simulink model "Sailboat_Modeling"  (R2024a)
settings: Solver=VariableStepAuto  StartTime=0.0  StopTime=10.0  RelTol=1e-3
values from neighbouring files (symbols this model uses):
  Ixx = 1/120 * pi * rho * L * B * T * (4*T^2 + B^2)    (= 0.835683076278)    [parameterCalculations.m]
  Izz = 1/120 * pi * rho * L * B * T * (B^2 + L^2)    (= 1.17027496573)    [parameterCalculations.m]
  m = 2.7    [parameterCalculations.m]
  m11 = m*k11    [parameterCalculations.m]
  m22 = m*k22    [parameterCalculations.m]
  m24 = 0    [parameterCalculations.m]
  m26 = xb*m22    [parameterCalculations.m]
  m66 = k66*Izz    [parameterCalculations.m]
  Nr = -pi * T^2/L^2 * (0.25 +0.039 * B/T - 0.56 * B/L)    (= -0.104988463049)    [parameterCalculations.m]
  Nv = -pi * T^2/L^2 * (0.5 +2.4 * T/L)    (= -0.841300100031)    [parameterCalculations.m]
  Yv = -pi * T^2/L^2 * (1 +0.4 * CB * B/T)    (= -0.560439243466)    [parameterCalculations.m]
libraries: cstblocks x4, simulink x3, vrlib x1
settings Model: Creator=Ruben  LastModifiedBy=Ruben

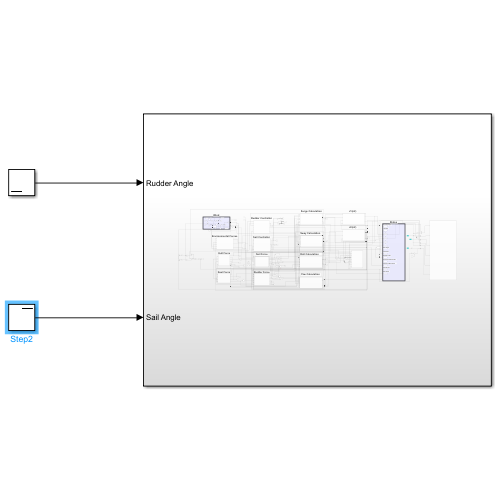
[thumbnail: Simulink's stored preview of the top-level diagram]
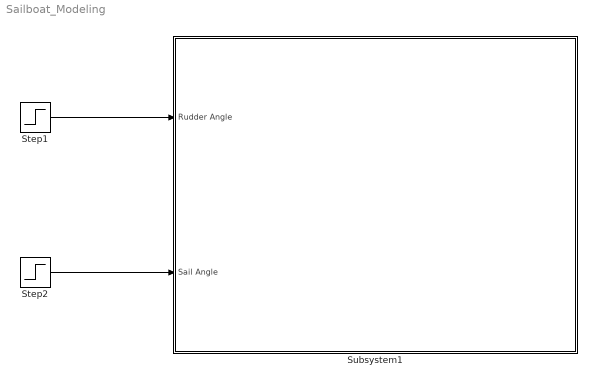
== system Sailboat_Modeling ==
  Step1 : Step  Time=0  After=0  SampleTime=0
  Step2 : Step  Time=0  After=pi/4  SampleTime=0
  Subsystem1 : Subsystem
  wires:
  Step2/1 -> Subsystem1/2(Sail Angle)
  Step1/1 -> Subsystem1/1(Rudder Angle)

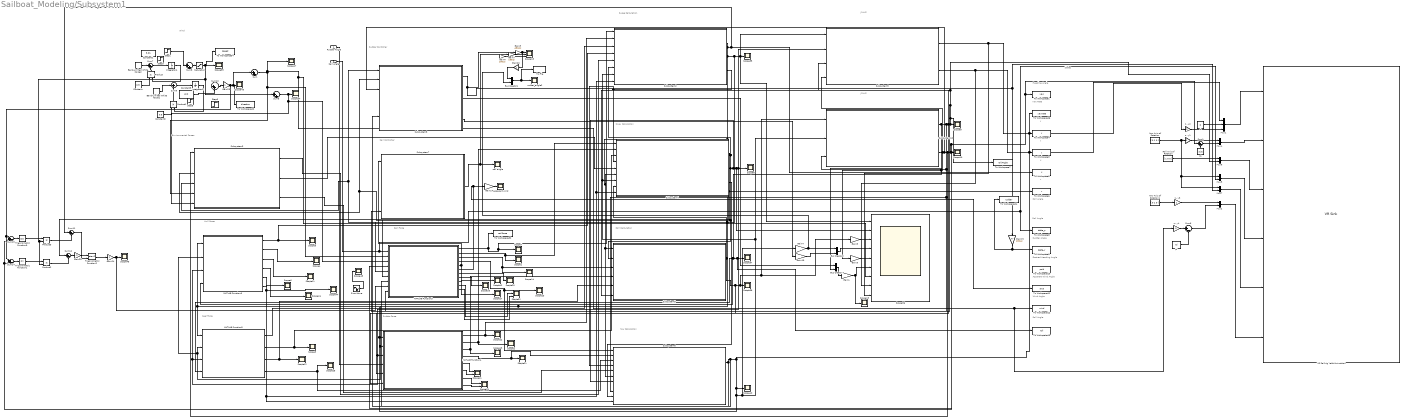
== system Sailboat_Modeling/Subsystem1 ==
  note: Keel Force
  note: Rudder Force
  note: Wind
  note: Sway Calculation
  note: Desired Heading Angle
  note: Sail Force
  note: u
  note: Environmental Forces
  note: J1(n2)
  note: Rudder Angle
  note: Apparent Wind Angle
  note: Yaw Calculation
  note: y
  note: v
  note: Surge Calculation
  note: Rudder Controller
  note: Wind Angle
  note: x
  note: States
  note: Heading Angle
  note: Sail Angle
  note: J2(n2)
  note: Sail Controller
  note: Yaw Rate
  note: Hull Force
  note: Roll Calculation
  note: Roll Angle
  note: Roll Angle
  Rudder Angle : Inport
  Sail Angle : Inport  Port=2
  Band-Limited White Noise1 : simulink/Sources/Band-Limited White Noise  Cov=[0.225]  Ts=0.01  seed=[3341]
  Band-Limited White Noise2 : simulink/Sources/Band-Limited White Noise  Cov=[0.2]  Ts=0.01  seed=[23341]
  Bus Creator : BusCreator  Inputs=2
  Bus Creator1 : BusCreator  Inputs=2
  Bus Creator2 : BusCreator  Inputs=2
  Constant : Constant  Value=0.5
  Constant1 : Constant  Value=3.01
  Constant2 : Constant  Value=0.5
  Constant3 : Constant  Value=pi/2
  Gain{1,3..7,14,18..19} (9 alike) : Gain  Gain=180/pi
  Gain20 : Gain
  Gain23 : Gain
  Gain24 : Gain
  Gain25 : Gain  Gain=-1
  Gain8 : Gain  Gain=-180/pi
  Integrator2 : Integrator  LimitOutput=on  UpperSaturationLimit=99  LowerSaturationLimit=-99
  Integrator4 : Integrator
  MATLAB Function3 : MATLAB Function  TreatAsAtomicUnit=on
  MATLAB Function4 : MATLAB Function  TreatAsAtomicUnit=on
  MATLAB Function5 : MATLAB Function  TreatAsAtomicUnit=on
  MATLAB Function6 : MATLAB Function  TreatAsAtomicUnit=on
  Mux1 : Mux  Inputs=3
  Mux{2,4..7} (5 alike) : Mux  Inputs=2
  Product{,1..3} (4 alike) : Product
  Roll Axis of Rotation : Constant  Value=[ 1 0 0 ]
  Saturation : Saturate  UpperLimit=6  LowerLimit=0
  Scope{1..14,17,19..27,34..35,37..40,42..45,48} (35 alike) : Scope
  Scope15 : Scope  NumInputPorts=3
  Scope31 : Scope  NumInputPorts=2
  Scope32 : Scope  NumInputPorts=2
  Scope36 : Scope  NumInputPorts=9
  Scope41 : Scope  NumInputPorts=2
  Sine Wave : Sin  Amplitude=pi  SampleTime=0
  Step1 : Step  Time=0  After=2  SampleTime=0
  Step3 : Step  Time=10  After=0.5  SampleTime=0
  Step5 : Step  Time=40  After=0.5  SampleTime=0
  Step6 : Step  Time=30  After=0.5  SampleTime=0
  Subsystem10 : Subsystem
  Subsystem2 : Subsystem
  Subsystem3 : Subsystem
  Subsystem4 : Subsystem
  Subsystem5 : Subsystem
  Subsystem6 : Subsystem
  Subsystem7 : Subsystem
  Subsystem8 : Subsystem
  Subsystem9 : Subsystem
  Sum{,5,8,10} (4 alike) : Sum  Inputs=|++
  Sum1 : Sum  Inputs=|+-  SaturateOnIntegerOverflow=on
  Sum{6..7,9,11..12} (5 alike) : Sum  Inputs=|+-
  Sum13 : Sum  Inputs=|-+-
  Sum14 : Sum  Inputs=|-+-
  To File : ToFile  Filename=sim_step.mat  SaveFormat=Timeseries
  To Workspace1 : ToWorkspace  VariableName=yaw  SaveFormat=Timeseries  SampleTime=0.01
  To Workspace10 : ToWorkspace  VariableName=psid  SaveFormat=Timeseries  SampleTime=0.01
  To Workspace11 : ToWorkspace  VariableName=awa  SaveFormat=Timeseries  SampleTime=-1
  To Workspace12 : ToWorkspace  VariableName=wind  SaveFormat=Timeseries  SampleTime=-1
  To Workspace13 : ToWorkspace  VariableName=roll  SaveFormat=Timeseries  SampleTime=-1
  To Workspace22 : ToWorkspace  VariableName=direction  SaveFormat=Timeseries  SampleTime=-1
  To Workspace24 : ToWorkspace  VariableName=rudder  SaveFormat=Timeseries  SampleTime=0.01
  To Workspace26 : ToWorkspace  VariableName=yawrate  SaveFormat=Timeseries  SampleTime=0.01
  To Workspace3 : ToWorkspace  VariableName=x  SaveFormat=Timeseries  SampleTime=-1
  To Workspace32 : ToWorkspace  VariableName=sailforce  SaveFormat=Timeseries  SampleTime=0.01
  To Workspace34 : ToWorkspace  VariableName=speed  SaveFormat=Timeseries  SampleTime=0.01
  To Workspace4 : ToWorkspace  VariableName=y  SaveFormat=Timeseries  SampleTime=-1
  To Workspace5 : ToWorkspace  VariableName=u  SaveFormat=Timeseries  SampleTime=0.01
  To Workspace6 : ToWorkspace  VariableName=v  SaveFormat=Timeseries  SampleTime=-1
  To Workspace7 : ToWorkspace  VariableName=rollAngle  SaveFormat=Timeseries  SampleTime=0.01
  To Workspace8 : ToWorkspace  VariableName=delta_s  SaveFormat=Timeseries  SampleTime=-1
  To Workspace9 : ToWorkspace  VariableName=delta_r  SaveFormat=Timeseries  SampleTime=0.01
  Trigonometric Function1 : Trigonometry
  Trigonometric Function2 : Trigonometry  Operator=atan2
  Trigonometric Function9 : Trigonometry  Operator=cos
  VR Sailing Yacht Animation : vrlib/VR Sink  InstantiateOnLoad=on  SampleTime=0.05  ViewEnable=on  RemoteChange=off  RemoteView=off  FieldsWritten=Hull_EarthFixed.translation.3.1.1.double#Rot_Yaw.rotation.4.1.1.double#Rot_Roll.rotation.4.1.1.double#Sail.rotation.4.1.1.double#Rudder.rotation.4.1.1.double#Wind_Arrow.rotation.4.1.1.double  WorldFileName=SailingYachtAnimation.wrl  WorldDescription=Sailing Yacht VR animation  AutoView=on  VideoDimensions=[]  AllowVariableSize=off  FigureProperties="{'Position', 'Name', 'Viewpoint', 'CameraBound', 'CameraDirection', 'CameraPosition', 'CameraUpVector', 'ZoomFactor', 'Antialiasing', 'Headlight', 'Lighting', 'Sound', 'StatusBar', 'Stereo3D', 'Stereo3DCameraOffset', 'Stereo3DHIT', 'ToolBar', 'Textures', 'Transparency', 'Triad', 'Wireframe', 'NavZones', 'NavMode', 'NavSpeed', 'CaptureFileFormat', 'CaptureFileName', 'Record2DCompressMethod', 'Record2DCompressQuality', 'Record2D', 'Record2DFileName', 'Record2DFPS', 'NavPanel'; [9.6200000000000000e+02   8.4000000000000000e+01   9.5800000000000000e+02   3.8000000000000000e+02], 'Sailing Yacht VR animation', 'Stern', 'on', [1.8779174371111376e-01  -8.0146307062595545e-01  -5.6779503997195024e-01], [-1.3398952830018864e+01   3.3896676016628582e+01   3.0405778585208221e+01], [8.9478754028877491e-02   5.8963553407129154e-01  -8.0269763269733285e-01], [1.0000000000000000e+00], 'on', 'on', 'on', 'on', 'on', 'off', [1.0000000149011612e-01], [0.0000000000000000e+00], 'on', 'on', 'on', 'none', 'off', 'off', 'fly', 'normal', 'tif', '%f_anim_%n.tif', 'auto', [7.5000000000000000e+01], 'off', '%f_anim_%n.avi', 'auto', 'halfbar'}"
  Yaw Axis of Rotation : Constant  Value=[ 0 1 0 ]
  Yaw Axis of Rotation1 : Constant  Value=[ 0 1 0 ]
  apparent wind : Scope
  pi : Constant  Value=-pi
  rudder_angle2 : Scope
  sail angle : Scope
  z : Constant  Value=0
  z - y1 : Gain
  z - y2 : Gain  Gain=-1
  z - y3 : Gain
  z - y4 : Gain  Gain=-1
  z1 : Constant  Value=pi/2
  wires:
  Step1/1 -> Sum8/1
  Bus Creator2/1 -> Scope36/4
  MATLAB Function3/2(Ys) -> Scope1/1, Subsystem4/1(sail force (Ys))
  Constant2/1 -> Product1/1
  Subsystem10/1(Phi) -> Gain3/1, MATLAB Function5/4(phi), MATLAB Function6/4(phi), To Workspace13/1, Scope37/1, Subsystem6/9(roll), Subsystem7/4(roll_angle), Subsystem10/3(phi), MATLAB Function4/6(phi), Subsystem9/3(phi), Scope9/1, To Workspace7/1, MATLAB Function3/9(phi), Subsystem5/6(rudder force (Kr)), Mux6/2
  Subsystem8/2(Desired Heading) -> Bus Creator/1
  Bus Creator1/1 -> To File/1, rudder_angle2/1
  Gain20/1 -> Bus Creator1/1
  Sum10/1 -> Gain23/1
  MATLAB Function6/1(Xh) -> Scope5/1, Subsystem2/4(hull force (Xh))
  MATLAB Function3/1(Xs) -> Subsystem2/1(sail force (Xs)), Scope7/1, To Workspace32/1
  MATLAB Function4/4(Nr) -> Scope21/1, Subsystem6/2(rudder force (Nr))
  MATLAB Function3/11(D) -> Scope32/2
  Subsystem7/1(sail angle) -> Gain7/1, sail angle/1
  Gain8/1 -> Gain20/1, Scope15/1
  Subsystem6/1(r) -> Subsystem8/6(r), To Workspace26/1, MATLAB Function5/1(r), MATLAB Function6/1(r), MATLAB Function4/1(r), Gain4/1, Subsystem10/2(r), Subsystem2/7(r), Subsystem4/7(r), Scope40/1, MATLAB Function3/7(r)
  MATLAB Function3/5(awa) -> Scope42/1, Subsystem7/1(apparent_wind_angle)
  MATLAB Function3/7(apparent_velocity) -> Scope20/1
  Gain19/1 -> Bus Creator2/2
  Subsystem8/3(desired yaw rate) -> Gain19/1
  Gain7/1 -> Scope15/2
  Gain1/1 -> Scope19/1, Scope36/6
  MATLAB Function5/2(Yk) -> Scope3/1, Subsystem4/3(keel force (Yk))
  MATLAB Function5/1(Xk) -> Subsystem2/3(keel force (Xk))
  Sum5/1 -> Scope34/1, Subsystem3/6(wind Velocity), MATLAB Function3/3(wind_velocity)
  Gain6/1 -> Scope15/3
  z/1 -> Mux1/2
  MATLAB Function4/7(lift_force) -> Scope31/1
  MATLAB Function3/10(L) -> Scope32/1
  Mux1/1 -> VR Sailing Yacht Animation/1
  Subsystem3/3(Ne) -> Subsystem6/5(environmental force (Ne))
  MATLAB Function3/9(V_awv) -> Scope27/1
  Subsystem4/2(v dot) -> Subsystem6/10(vdot)
  MATLAB Function3/8(V_awu) -> Scope26/1
  Subsystem9/1(x) -> Scope36/9, z - y2/1, To Workspace4/1
  MATLAB Function4/5(delta_r) -> Scope41/1
  MATLAB Function3/6(alpha_aw) -> To Workspace11/1, Gain14/1
  z1/1 -> Sum1/2
  MATLAB Function4/2(Yr) -> Scope2/1, Subsystem4/2(rudder force (Yr))
  Gain4/1 -> Bus Creator2/1, Bus Creator1/2
  Gain18/1 -> To Workspace9/1, To Workspace24/1
  MATLAB Function6/3(Kh) -> Scope11/1
  MATLAB Function3/3(Ks) -> Scope14/1, Subsystem5/3(sail force (Ks))
  MATLAB Function5/4(Nk) -> Scope25/1, Subsystem6/3(keel force (Nk))
  MATLAB Function4/3(Kr) -> Scope13/1, Subsystem5/4(roll angle)
  MATLAB Function5/3(Kk) -> Scope12/1, Subsystem5/5(keel force (Kk))
  Subsystem4/1(v) -> To Workspace6/1, MATLAB Function3/6(v), Subsystem2/6(v), Subsystem6/7(v), Scope36/2, Scope8/1, Subsystem9/2(v), MATLAB Function6/3(v), MATLAB Function5/3(v), MATLAB Function4/3(v), Subsystem5/2(v), Subsystem8/2(v), Subsystem3/3(v), Sum12/1
  MATLAB Function4/1(Xr) -> Subsystem2/2(rudder force (Xr)), Scope22/1
  Mux6/1 -> VR Sailing Yacht Animation/3
  Subsystem3/2(Ye) -> Subsystem4/5(environmental force (Ye))
  Subsystem3/1(Xe) -> Subsystem2/5(environmental force (Xe))
  Mux7/1 -> VR Sailing Yacht Animation/5
  Sine Wave/1 -> Scope48/1
  Subsystem10/2(Psi) -> Bus Creator/2, Subsystem9/4(psi), Sum14/2, Sum13/2, Sum1/1, To Workspace1/1, MATLAB Function3/4(psi), Scope10/1, Subsystem3/1(psi), Subsystem8/3(psi)
  Yaw Axis of Rotation/1 -> Mux5/1, Mux7/1, z - y1/1
  Constant3/1 -> Sum10/2
  z - y4/1 -> Sum6/1
  MATLAB Function6/4(Nh) -> Scope24/1
  MATLAB Function4/6(alpha_a) -> Scope41/2
  z - y3/1 -> Mux2/1
  Subsystem8/1(rudder angle) -> Gain8/1, Gain18/1, Mux7/2
  Subsystem5/1(p) -> MATLAB Function4/5(p), Subsystem10/1(p), Gain5/1, Scope38/1, Subsystem4/8(p)
  Saturation/1 -> Product2/2, Product3/2, Sum5/1, Scope39/1, To Workspace34/1
  MATLAB Function4/8(drag_force) -> Scope31/2
  Sum6/1 -> Mux2/2
  MATLAB Function6/2(Yh) -> Scope4/1
  Integrator2/1 -> Product1/2
  Band-Limited White Noise1/1 -> Sum9/1
  MATLAB Function3/4(Ns) -> Subsystem6/1(sail force (Ns)), Scope23/1
  Integrator4/1 -> Product/2
  MATLAB Function6/6(alpha_ah) -> Subsystem6/11(hull_ah), Subsystem2/8(hull_ah), Subsystem4/9(hull_ah), Scope44/1
  Sum/1 -> Scope17/1, Scope36/7, z - y4/1, To Workspace12/1, MATLAB Function3/2(wind_direction), Subsystem3/5(wind Direction)
  Product1/1 -> Sum9/2
  Band-Limited White Noise2/1 -> Sum7/1
  Product/1 -> Sum7/2
  Subsystem2/1(u) -> MATLAB Function5/2(u), MATLAB Function6/2(u), MATLAB Function4/2(u), Subsystem8/1(u), Subsystem3/4(u), Subsystem6/6(u), Subsystem5/1(u), Subsystem4/6(u), MATLAB Function3/5(u), Scope36/1, Subsystem9/1(u), Scope35/1, Sum11/1, To Workspace5/1
  Sum7/1 -> Integrator4/1
  z - y1/1 -> Mux4/1
  pi/1 -> Sum6/2
  Sum9/1 -> Integrator2/1
  Mux4/1 -> VR Sailing Yacht Animation/2
  Bus Creator/1 -> Gain1/1
  Gain14/1 -> apparent wind/1
  Gain5/1 -> Scope36/3
  Constant/1 -> Product/1
  Gain23/1 -> Sum14/1, Sum13/1, Sum/1, To Workspace22/1, Scope43/1
  Subsystem9/2(y) -> Scope36/8, Mux1/1, To Workspace3/1
  Subsystem2/2(hull) -> Subsystem6/4(hull force (Nh)), Subsystem4/4("hull force ")
  Yaw Axis of Rotation1/1 -> z - y3/1
  MATLAB Function6/5(Frh) -> Scope6/1
  Sum1/1 -> Mux4/2
  Gain3/1 -> Scope36/5
  Mux5/1 -> VR Sailing Yacht Animation/4
  Sum8/1 -> Saturation/1
  Mux2/1 -> VR Sailing Yacht Animation/6
  Roll Axis of Rotation/1 -> Mux6/1
  z - y2/1 -> Mux1/3
  Rudder Angle/1 -> MATLAB Function4/4("delta_r ")
  Product2/1 -> Sum12/2
  Gain25/1 -> Trigonometric Function2/1
  Gain24/1 -> MATLAB Function3/8(rawa), Scope45/1
  Sum12/1 -> Gain25/1
  Sum13/1 -> Trigonometric Function9/1
  Sum14/1 -> Trigonometric Function1/1
  Product3/1 -> Sum11/2
  Trigonometric Function1/1 -> Product2/1
  Trigonometric Function9/1 -> Product3/1
  Trigonometric Function2/1 -> Gain24/1
  Sum11/1 -> Trigonometric Function2/2
  Sail Angle/1 -> To Workspace8/1, Mux5/2, MATLAB Function3/1(delta_s)

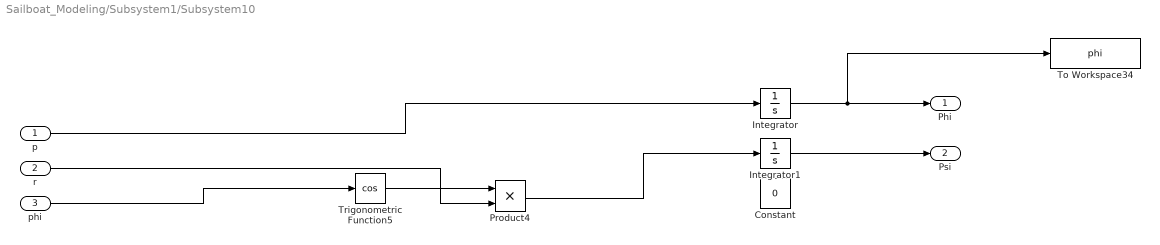
== system Sailboat_Modeling/Subsystem1/Subsystem10 ==
  p : Inport
  r : Inport  Port=2
  phi : Inport  Port=3
  Constant : Constant  Value=0
  Integrator : Integrator
  Integrator1 : Integrator
  Product4 : Product
  To Workspace34 : ToWorkspace  VariableName=phi  SaveFormat=Timeseries  SampleTime=0.01
  Trigonometric Function5 : Trigonometry  Operator=cos
  Phi : Outport
  Psi : Outport  Port=2
  wires:
  Integrator/1 -> To Workspace34/1, Phi/1
  p/1 -> Integrator/1
  Trigonometric Function5/1 -> Product4/1
  Product4/1 -> Integrator1/1
  r/1 -> Product4/2
  phi/1 -> Trigonometric Function5/1
  Integrator1/1 -> Psi/1

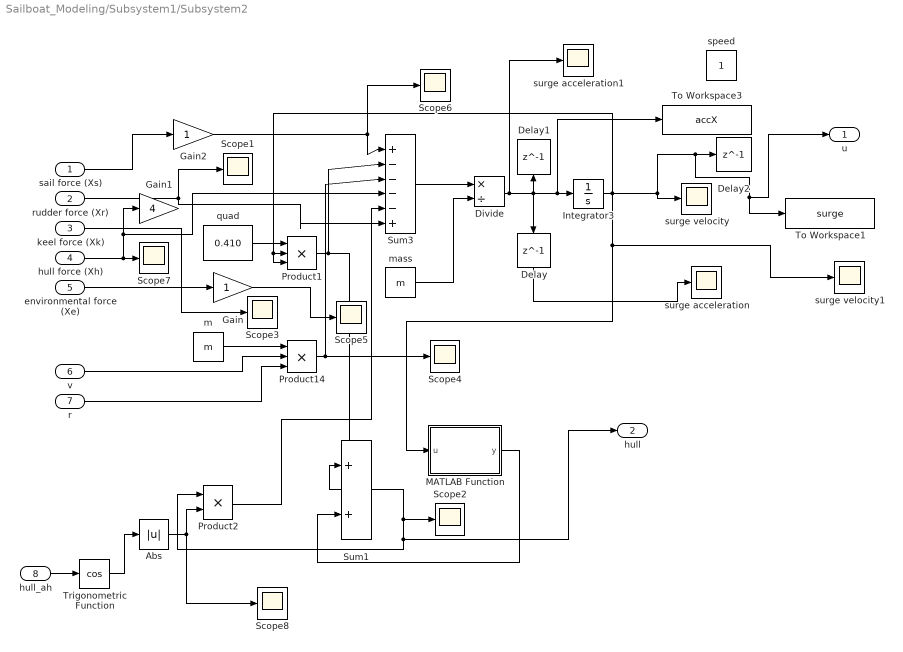
== system Sailboat_Modeling/Subsystem1/Subsystem2 ==
  sail force (Xs) : Inport
  rudder force (Xr) : Inport  Port=2
  keel force (Xk) : Inport  Port=3
  hull force (Xh) : Inport  Port=4
  environmental force (Xe) : Inport  Port=5
  v : Inport  Port=6
  r : Inport  Port=7
  hull_ah : Inport  Port=8
  Abs : Abs  SaturateOnIntegerOverflow=off
  Delay : Delay  DelayLength=1  InitialCondition=0
  Delay1 : Delay  DelayLength=1  InitialCondition=0
  Delay2 : Delay  DelayLength=1  InitialCondition=0
  Divide : Product  Inputs=*/
  Gain : Gain
  Gain1 : Gain  Gain=4
  Gain2 : Gain
  Integrator3 : Integrator  InitialCondition=1  LimitOutput=on  UpperSaturationLimit=1.5  LowerSaturationLimit=0
  MATLAB Function : MATLAB Function  TreatAsAtomicUnit=on
  Product1 : Product  Inputs=3
  Product14 : Product  Inputs=3
  Product2 : Product
  Scope{1..8} (8 alike) : Scope
  Sum1 : Sum  Inputs=|++
  Sum3 : Sum  Inputs=|+----+
  To Workspace1 : ToWorkspace  VariableName=surge  SaveFormat=Timeseries  SampleTime=0.01
  To Workspace3 : ToWorkspace  VariableName=accX  SaveFormat=Timeseries  SampleTime=-1
  Trigonometric Function : Trigonometry  Operator=cos
  m : Constant  Value=m
  mass : Constant  Value=m
  quad : Constant  Value=0.410
  speed : Constant
  surge acceleration : Scope
  surge acceleration1 : Scope
  surge velocity : Scope
  surge velocity1 : Scope
  u : Outport
  hull : Outport  Port=2
  wires:
  m/1 -> Product14/1
  mass/1 -> Divide/2
  Sum3/1 -> Divide/1
  rudder force (Xr)/1 -> Sum3/6, Scope1/1
  keel force (Xk)/1 -> Scope3/1
  environmental force (Xe)/1 -> Gain/1
  r/1 -> Product14/3
  v/1 -> Product14/2
  Delay/1 -> surge acceleration/1
  Divide/1 -> Delay/1, Delay1/1, To Workspace3/1, Integrator3/1, surge acceleration1/1
  quad/1 -> Product1/1
  hull force (Xh)/1 -> Sum3/4, Gain1/1, Scope7/1
  Product14/1 -> Sum3/3, Scope4/1
  Gain/1 -> Scope5/1
  Product1/1 -> Sum1/1, Sum3/2
  sail force (Xs)/1 -> Gain2/1
  MATLAB Function/1(y) -> Sum1/2
  hull_ah/1 -> Trigonometric Function/1
  Trigonometric Function/1 -> Abs/1
  Sum1/1 -> hull/1, Product2/1, Scope2/1
  Product2/1 -> Sum3/5
  Abs/1 -> Scope8/1, Product2/2
  Integrator3/1 -> Product1/3, Product1/2, MATLAB Function/1(u), surge velocity1/1, u/1, To Workspace1/1, Delay2/1, surge velocity/1
  Gain2/1 -> Scope6/1, Sum3/1

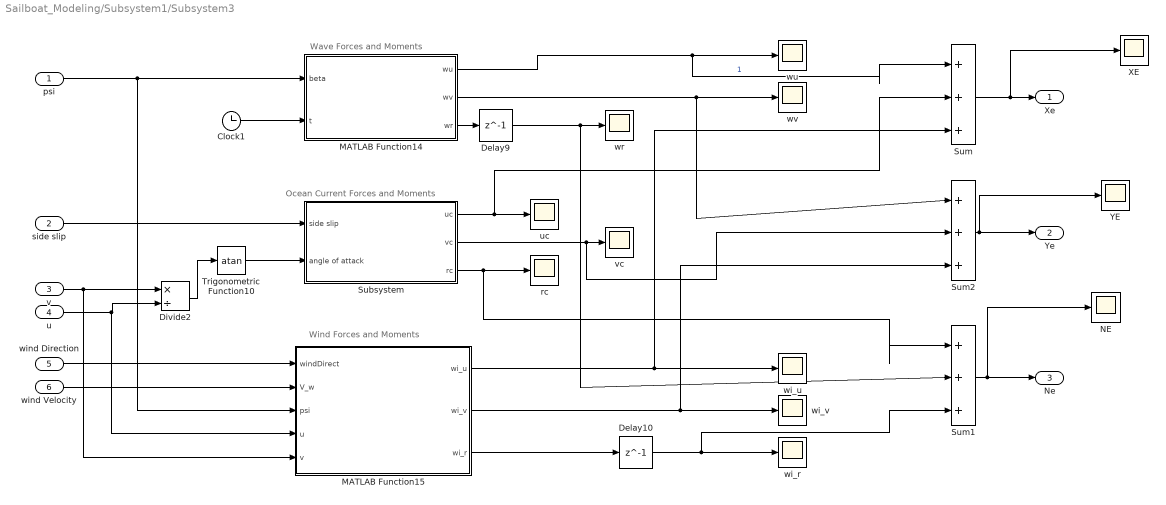
== system Sailboat_Modeling/Subsystem1/Subsystem3 ==
  note: Wave Forces and Moments
  note: Wind Forces and Moments
  note: Ocean Current Forces and Moments
  psi : Inport
  side slip : Inport  Port=2
  v : Inport  Port=3
  u : Inport  Port=4
  wind Direction : Inport  Port=5
  wind Velocity : Inport  Port=6
  Clock1 : Clock
  Delay10 : Delay  DelayLength=1
  Delay9 : Delay  DelayLength=1
  Divide2 : Product  Inputs=*/
  MATLAB Function14 : MATLAB Function  TreatAsAtomicUnit=on
  MATLAB Function15 : MATLAB Function  TreatAsAtomicUnit=on
  NE : Scope
  Subsystem : Subsystem
  Sum : Sum  Inputs=|+++
  Sum1 : Sum  Inputs=|+++
  Sum2 : Sum  Inputs=|+++
  Trigonometric Function10 : Trigonometry  Operator=atan
  XE : Scope
  YE : Scope
  rc : Scope
  uc : Scope
  vc : Scope
  wi_r : Scope
  wi_u : Scope
  wi_v : Scope
  wr : Scope
  wu : Scope
  wv : Scope
  Xe : Outport
  Ye : Outport  Port=2
  Ne : Outport  Port=3
  wires:
  MATLAB Function14/2(wv) -> Sum2/1, wv/1
  Trigonometric Function10/1 -> Subsystem/2(angle of attack)
  MATLAB Function14/3(wr) -> Delay9/1
  MATLAB Function15/2(wi_v) -> Sum2/3, wi_v/1
  Subsystem/1(uc) -> Sum/2, uc/1
  MATLAB Function15/3(wi_r) -> Delay10/1
  MATLAB Function15/1(wi_u) -> Sum/3, wi_u/1
  Clock1/1 -> MATLAB Function14/2(t)
  Subsystem/2(vc) -> Sum2/2, vc/1
  MATLAB Function14/1(wu) -> Sum/1, wu/1  "1"
  Divide2/1 -> Trigonometric Function10/1
  psi/1 -> MATLAB Function14/1(beta), MATLAB Function15/3(psi)
  side slip/1 -> Subsystem/1(side slip)
  v/1 -> MATLAB Function15/5(v), Divide2/1
  u/1 -> MATLAB Function15/4(u), Divide2/2
  wind Direction/1 -> MATLAB Function15/1(windDirect)
  wind Velocity/1 -> MATLAB Function15/2(V_w)
  Delay10/1 -> Sum1/3, wi_r/1
  Subsystem/3(rc) -> Sum1/1, rc/1
  Delay9/1 -> Sum1/2, wr/1
  Sum/1 -> XE/1, Xe/1
  Sum1/1 -> NE/1, Ne/1
  Sum2/1 -> YE/1, Ye/1

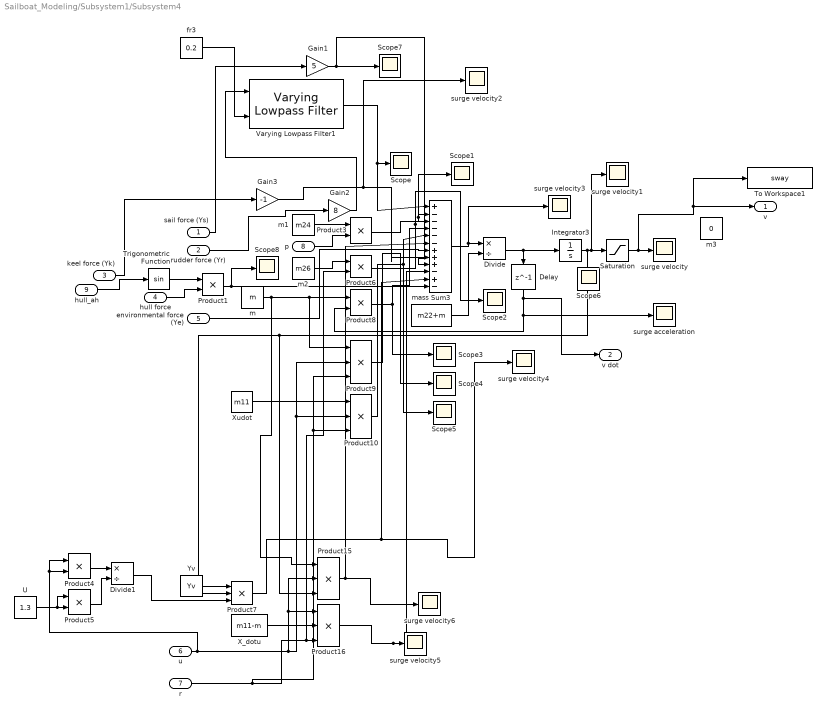
== system Sailboat_Modeling/Subsystem1/Subsystem4 ==
  sail force (Ys) : Inport
  rudder force (Yr) : Inport  Port=2
  keel force (Yk) : Inport  Port=3
  "hull force " : Inport  Port=4
  environmental force (Ye) : Inport  Port=5
  u : Inport  Port=6
  r : Inport  Port=7
  p : Inport  Port=8
  hull_ah : Inport  Port=9
  Delay : Delay  DelayLength=1  InitialCondition=0
  Divide : Product  Inputs=*/
  Divide1 : Product  Inputs=*/
  Gain1 : Gain  Gain=5
  Gain2 : Gain  Gain=8
  Gain3 : Gain  Gain=-1
  Integrator3 : Integrator  UpperSaturationLimit=0.01  LowerSaturationLimit=-0.01
  Product{1,3..6,8} (6 alike) : Product
  Product{7,9..10,15..16} (5 alike) : Product  Inputs=3
  Saturation : Saturate  UpperLimit=0.4  LowerLimit=-0.4
  Scope{,1..8} (9 alike) : Scope
  Sum3 : Sum  Inputs=|+-----+++-+-
  To Workspace1 : ToWorkspace  VariableName=sway  SaveFormat=Timeseries  SampleTime=0.01
  Trigonometric Function : Trigonometry
  U : Constant  Value=1.3
  Varying Lowpass Filter1 : cstblocks/Linear Parameter Varying/Varying Lowpass Filter  N=1
  X_dotu : Constant  Value=m11-m
  Xudot : Constant  Value=m11
  Yv : Constant  Value=Yv
  fr3 : Constant  Value=0.2
  m : Constant  Value=m
  m1 : Constant  Value=m24
  m2 : Constant  Value=m26
  m3 : Constant  Value=0
  mass : Constant  Value=m22+m
  surge acceleration : Scope
  surge velocity{,1..6} (7 alike) : Scope
  v : Outport
  v dot : Outport  Port=2
  wires:
  sail force (Ys)/1 -> Gain1/1
  mass/1 -> Divide/2
  Sum3/1 -> surge velocity3/1, Divide/1
  X_dotu/1 -> Product16/2
  Yv/1 -> Product7/1
  Product15/1 -> surge velocity6/1, Sum3/6
  Product16/1 -> surge velocity5/1, Sum3/10
  r/1 -> Product10/3, Product9/3, Product6/2, Product16/3
  fr3/1 -> Varying Lowpass Filter1/2
  Varying Lowpass Filter1/1 -> Scope/1, Sum3/1
  keel force (Yk)/1 -> Gain3/1
  Product5/1 -> Divide1/2
  U/1 -> Product5/1, Product5/2
  Product4/1 -> Divide1/1
  Divide1/1 -> Product7/3
  Integrator3/1 -> surge velocity1/1, Saturation/1, Product15/3, Product7/2
  m1/1 -> Product3/1
  Product3/1 -> Scope1/1, Sum3/2
  Product6/1 -> Scope2/1, Sum3/3
  m2/1 -> Product6/1
  Product8/1 -> Sum3/4, Scope3/1
  m/1 -> Product15/1, Product9/1, Product8/1
  u/1 -> Product10/2, Product9/2, Product16/1, Product15/2, Product4/1, Product4/2
  Xudot/1 -> Product10/1
  rudder force (Yr)/1 -> Gain2/1
  Product9/1 -> Scope4/1
  Product10/1 -> Sum3/5, Scope5/1
  Gain1/1 -> Sum3/9, Scope7/1
  Gain3/1 -> Sum3/8, surge velocity2/1
  p/1 -> Product3/2
  Saturation/1 -> v/1, To Workspace1/1, surge velocity/1
  environmental force (Ye)/1 -> Sum3/7
  Product7/1 -> Sum3/11, surge velocity4/1
  Divide/1 -> Delay/1, Integrator3/1
  Delay/1 -> v dot/1, Product8/2, surge acceleration/1
  "hull force "/1 -> Product1/2
  Product1/1 -> Scope8/1, Sum3/12
  Trigonometric Function/1 -> Product1/1
  hull_ah/1 -> Trigonometric Function/1
  Gain2/1 -> Varying Lowpass Filter1/1

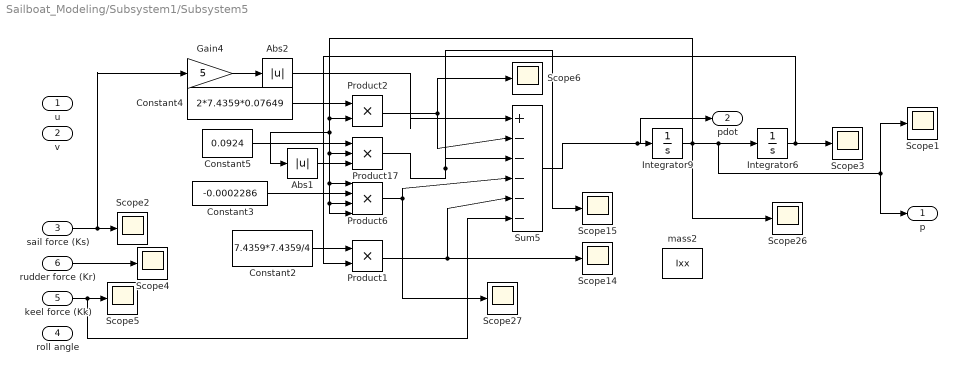
== system Sailboat_Modeling/Subsystem1/Subsystem5 ==
  u : Inport
  v : Inport  Port=2
  sail force (Ks) : Inport  Port=3
  roll angle : Inport  Port=4
  keel force (Kk) : Inport  Port=5
  rudder force (Kr) : Inport  Port=6
  Abs1 : Abs  SaturateOnIntegerOverflow=off
  Abs2 : Abs  SaturateOnIntegerOverflow=off
  Constant2 : Constant  Value=7.4359*7.4359/4
  Constant3 : Constant  Value=-0.0002286
  Constant4 : Constant  Value=2*7.4359*0.07649
  Constant5 : Constant  Value=0.0924
  Gain4 : Gain  Gain=5
  Integrator6 : Integrator
  Integrator9 : Integrator
  Product1 : Product
  Product17 : Product  Inputs=3
  Product2 : Product
  Product6 : Product  Inputs=4
  Scope{1..6,14..15,26..27} (10 alike) : Scope
  Sum5 : Sum  Inputs=|+-----
  mass2 : Constant  Value=Ixx
  p : Outport
  pdot : Outport  Port=2
  wires:
  Integrator9/1 -> Scope26/1, Product6/1, Product6/4, Product6/3, Product17/2, Abs1/1, Product2/2, Scope1/1, p/1, Integrator6/1
  Constant3/1 -> Product6/2
  Product2/1 -> Sum5/2, Scope6/1
  Sum5/1 -> pdot/1, Integrator9/1
  sail force (Ks)/1 -> Gain4/1, Scope2/1
  Constant4/1 -> Product2/1
  Abs1/1 -> Product17/3
  Constant5/1 -> Product17/1
  Constant2/1 -> Product1/1
  Product1/1 -> Sum5/5, Scope14/1
  Product6/1 -> Scope27/1, Sum5/4
  Product17/1 -> Scope15/1, Sum5/3
  Integrator6/1 -> Product1/2, Scope3/1
  rudder force (Kr)/1 -> Scope4/1
  keel force (Kk)/1 -> Sum5/6, Scope5/1
  Gain4/1 -> Abs2/1
  Abs2/1 -> Sum5/1

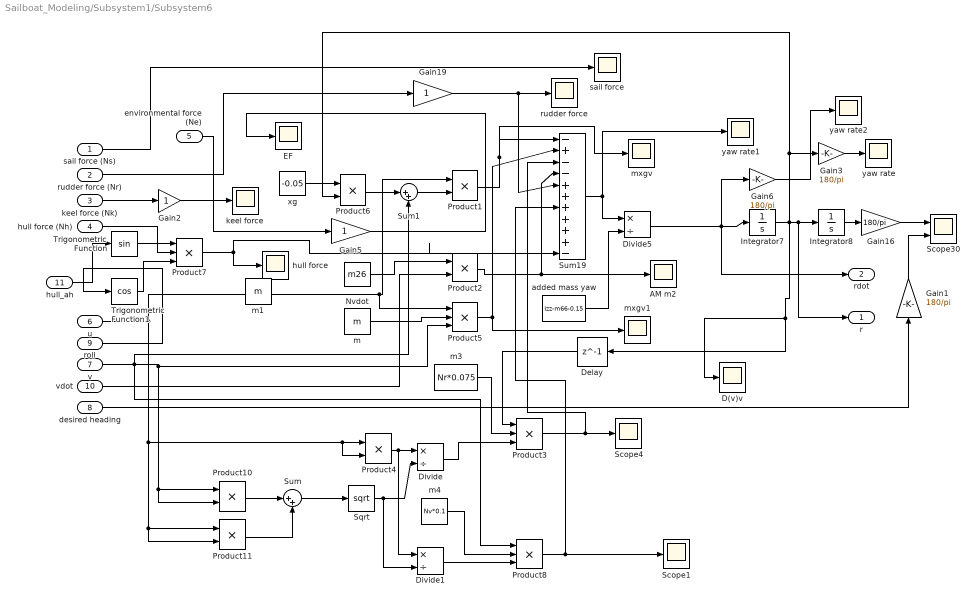
== system Sailboat_Modeling/Subsystem1/Subsystem6 ==
  sail force (Ns) : Inport
  rudder force (Nr) : Inport  Port=2
  keel force (Nk) : Inport  Port=3
  hull force (Nh) : Inport  Port=4
  environmental force (Ne) : Inport  Port=5
  u : Inport  Port=6
  v : Inport  Port=7
  desired heading : Inport  Port=8
  roll : Inport  Port=9
  vdot : Inport  Port=10
  hull_ah : Inport  Port=11
  AM m2 : Scope
  D(v)v : Scope
  Delay : Delay  DelayLength=1  InitialCondition=0
  Divide : Product  Inputs=*/
  Divide1 : Product  Inputs=*/
  Divide5 : Product  Inputs=*/
  EF : Scope
  Gain{1,3,6,16} (4 alike) : Gain  Gain=180/pi
  Gain19 : Gain
  Gain2 : Gain
  Gain5 : Gain
  Integrator7 : Integrator
  Integrator8 : Integrator
  Nvdot : Constant  Value=m26
  Product{1..2,4,6,10..11} (6 alike) : Product
  Product{3,5,7..8} (4 alike) : Product  Inputs=3
  Scope1 : Scope
  Scope30 : Scope  NumInputPorts=2
  Scope4 : Scope
  Sqrt : Sqrt
  Sum : Sum  Inputs=|++
  Sum1 : Sum  Inputs=|++
  Sum19 : Sum  Inputs=|-+--++++++-
  Trigonometric Function : Trigonometry
  Trigonometric Function1 : Trigonometry  Operator=cos
  added mass yaw : Constant  Value=Izz-m66-0.15  VectorParams1D=off
  hull force : Scope
  keel force : Scope
  m : Constant  Value=m
  m1 : Constant  Value=m
  m3 : Constant  Value=Nr*0.075
  m4 : Constant  Value=Nv*0.1
  mxgv : Scope
  mxgv1 : Scope
  rudder force : Scope
  sail force : Scope
  xg : Constant  Value=-0.05
  yaw rate : Scope
  yaw rate1 : Scope
  yaw rate2 : Scope
  r : Outport
  rdot : Outport  Port=2
  wires:
  Gain16/1 -> Scope30/1
  added mass yaw/1 -> Divide5/2
  Sum19/1 -> Divide5/1, yaw rate1/1
  sail force (Ns)/1 -> sail force/1
  rudder force (Nr)/1 -> Gain19/1
  environmental force (Ne)/1 -> Gain5/1
  u/1 -> Product1/1, Product5/1, Product11/2, Product11/1, Product4/2, Product4/1
  Nvdot/1 -> Product2/1
  desired heading/1 -> Gain1/1
  Integrator8/1 -> Gain16/1
  Gain1/1 -> Scope30/2
  Gain19/1 -> Sum19/5, rudder force/1
  keel force (Nk)/1 -> Gain2/1
  Gain2/1 -> keel force/1
  Integrator7/1 -> r/1, Integrator8/1, Delay/1, D(v)v/1, Product6/2, Gain3/1
  m3/1 -> Product3/2
  Product4/1 -> Divide/1, Divide1/1
  Sqrt/1 -> Divide1/2, Divide/2
  vdot/1 -> Product2/2
  Product8/1 -> Sum19/7, Scope1/1
  Product3/1 -> Sum19/3, Scope4/1
  m/1 -> Product5/2
  Product1/1 -> Sum19/1, mxgv/1
  Divide/1 -> Product3/3
  Product10/1 -> Sum/1
  Product11/1 -> Sum/2
  v/1 -> Product8/1, Product5/3, Product10/2, Product10/1, Sum1/2
  Sum/1 -> Sqrt/1
  m4/1 -> Product8/2
  Divide1/1 -> Product8/3
  Product2/1 -> Sum19/4, AM m2/1
  Product6/1 -> Sum1/1
  xg/1 -> Product6/1
  Sum1/1 -> Product1/2
  Product5/1 -> mxgv1/1, Sum19/2
  Gain5/1 -> EF/1
  Gain6/1 -> yaw rate2/1
  Delay/1 -> Product3/1
  Divide5/1 -> Gain6/1, Integrator7/1, rdot/1
  hull force (Nh)/1 -> Product7/2
  Trigonometric Function/1 -> Product7/1
  hull_ah/1 -> Trigonometric Function/1
  Product7/1 -> hull force/1, Sum19/11
  roll/1 -> Trigonometric Function1/1
  Trigonometric Function1/1 -> Product7/3
  Gain3/1 -> yaw rate/1

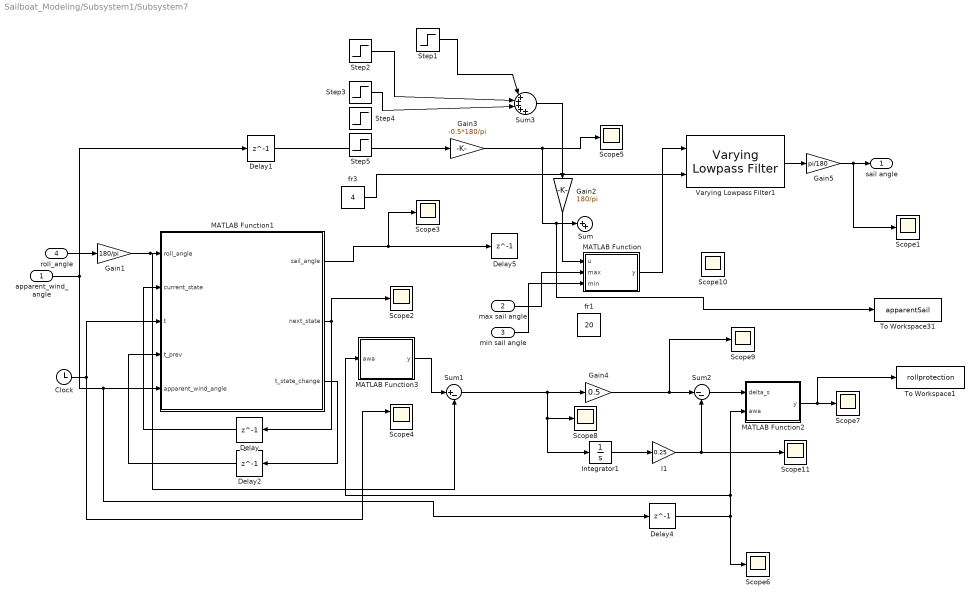
== system Sailboat_Modeling/Subsystem1/Subsystem7 ==
  apparent_wind_angle : Inport
  max sail angle : Inport  Port=2
  min sail angle : Inport  Port=3
  roll_angle : Inport  Port=4
  Clock : Clock
  Delay{,1..2,4..5} (5 alike) : Delay  DelayLength=1  InitialCondition=0
  Gain1 : Gain  Gain=180/pi
  Gain2 : Gain  Gain=180/pi
  Gain3 : Gain  Gain=-0.5*180/pi
  Gain4 : Gain  Gain=0.5
  Gain5 : Gain  Gain=pi/180
  I1 : Gain  Gain=0.25
  Integrator1 : Integrator
  MATLAB Function : MATLAB Function  TreatAsAtomicUnit=on
  MATLAB Function1 : MATLAB Function  TreatAsAtomicUnit=on
  MATLAB Function2 : MATLAB Function  TreatAsAtomicUnit=on
  MATLAB Function3 : MATLAB Function  TreatAsAtomicUnit=on
  Scope{1..3,5..11} (10 alike) : Scope
  Scope4 : Scope  NumInputPorts=2
  Step1 : Step  Time=0  After=80/180*pi  SampleTime=0
  Step2 : Step  Time=15  After=-35/180*pi  SampleTime=0
  Step3 : Step  Time=30  After=-30/180*pi  SampleTime=0
  Step4 : Step  Time=30  After=-pi/9  SampleTime=0
  Step5 : Step  Time=40  After=-pi/18  SampleTime=0
  Sum : Sum  Inputs=|++
  Sum1 : Sum  Inputs=|+-
  Sum2 : Sum  Inputs=|--
  Sum3 : Sum  Inputs=|+++++
  To Workspace1 : ToWorkspace  VariableName=rollprotection  SaveFormat=Timeseries  SampleTime=0.01
  To Workspace31 : ToWorkspace  VariableName=apparentSail  SaveFormat=Timeseries  SampleTime=0.01
  Varying Lowpass Filter1 : cstblocks/Linear Parameter Varying/Varying Lowpass Filter  N=1
  fr1 : Constant  Value=20
  fr3 : Constant  Value=4
  sail angle : Outport
  wires:
  fr3/1 -> Varying Lowpass Filter1/2
  max sail angle/1 -> MATLAB Function/2(max)
  min sail angle/1 -> MATLAB Function/3(min)
  MATLAB Function1/2(next_state) -> Scope2/1, Delay/1
  MATLAB Function1/3(t_state_change) -> Delay2/1
  Clock/1 -> Scope4/1, MATLAB Function1/3(t)
  Delay/1 -> MATLAB Function1/2(current_state)
  Delay2/1 -> MATLAB Function1/4(t_prev)
  MATLAB Function1/1(sail_angle) -> Scope3/1, Delay5/1
  apparent_wind_angle/1 -> Delay4/1, MATLAB Function1/5(apparent_wind_angle), Delay1/1
  roll_angle/1 -> Gain1/1
  Delay1/1 -> Gain3/1
  Gain3/1 -> To Workspace31/1, Sum/1, Scope5/1
  Gain1/1 -> Sum1/2, MATLAB Function1/1(roll_angle)
  Delay4/1 -> MATLAB Function3/1(awa), MATLAB Function2/2(awa), Scope6/1
  Varying Lowpass Filter1/1 -> Gain5/1
  MATLAB Function2/1(y) -> Scope7/1, To Workspace1/1
  Gain5/1 -> Scope1/1, sail angle/1
  Integrator1/1 -> I1/1
  I1/1 -> Scope11/1, Sum2/2
  Gain4/1 -> Scope9/1, Sum2/1
  Sum2/1 -> MATLAB Function2/1(delta_s)
  Sum1/1 -> Integrator1/1, Scope8/1, Gain4/1
  MATLAB Function/1(y) -> Varying Lowpass Filter1/1
  MATLAB Function3/1(y) -> Sum1/1
  Sum3/1 -> Gain2/1
  Step1/1 -> Sum3/1
  Gain2/1 -> MATLAB Function/1(u)
  Step2/1 -> Sum3/2
  Step3/1 -> Sum3/3

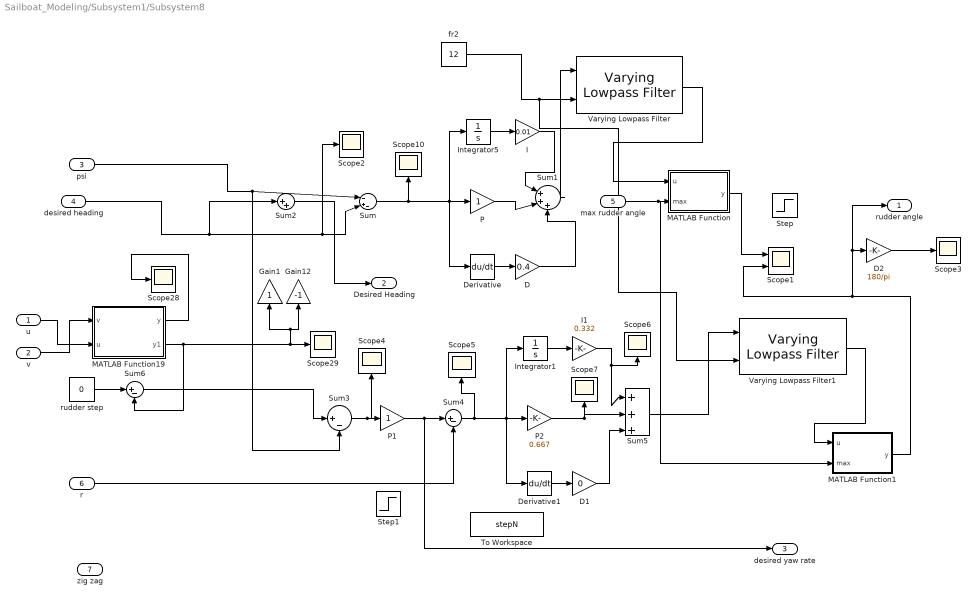
== system Sailboat_Modeling/Subsystem1/Subsystem8 ==
  u : Inport
  v : Inport  Port=2
  psi : Inport  Port=3
  desired heading : Inport  Port=4
  max rudder angle : Inport  Port=5
  r : Inport  Port=6
  zig zag : Inport  Port=7
  D : Gain  Gain=0.4
  D1 : Gain  Gain=0
  D2 : Gain  Gain=180/pi
  Derivative : Derivative
  Derivative1 : Derivative
  Gain1 : Gain
  Gain12 : Gain  Gain=-1
  I : Gain  Gain=0.01
  I1 : Gain  Gain=0.332
  Integrator1 : Integrator
  Integrator5 : Integrator
  MATLAB Function : MATLAB Function  TreatAsAtomicUnit=on
  MATLAB Function1 : MATLAB Function  TreatAsAtomicUnit=on
  MATLAB Function19 : MATLAB Function  TreatAsAtomicUnit=on
  P : Gain
  P1 : Gain
  P2 : Gain  Gain=0.667
  Scope1 : Scope  NumInputPorts=2
  Scope{2..7,10,28..29} (9 alike) : Scope
  Step : Step  Time=0.01  After=0.1945  SampleTime=0
  Step1 : Step  Time=5  After=0  SampleTime=0
  Sum : Sum  Inputs=|-+-
  Sum1 : Sum  Inputs=|+++
  Sum2 : Sum  Inputs=|++
  Sum3 : Sum  Inputs=|+-
  Sum4 : Sum  Inputs=|+-
  Sum5 : Sum  Inputs=|+++
  Sum6 : Sum  Inputs=|+-
  To Workspace : ToWorkspace  VariableName=stepN  SaveFormat=Timeseries  SampleTime=-1
  Varying Lowpass Filter : cstblocks/Linear Parameter Varying/Varying Lowpass Filter  N=1
  Varying Lowpass Filter1 : cstblocks/Linear Parameter Varying/Varying Lowpass Filter  N=1
  fr2 : Constant  Value=12
  rudder step : Constant  Value=0
  rudder angle : Outport
  Desired Heading : Outport  Port=2
  desired yaw rate : Outport  Port=3
  wires:
  Varying Lowpass Filter/1 -> MATLAB Function/1(u)
  MATLAB Function/1(y) -> Scope1/1
  Sum1/1 -> Varying Lowpass Filter/1
  I/1 -> Sum1/1
  Sum/1 -> Scope10/1, Derivative/1, Integrator5/1, P/1
  fr2/1 -> Varying Lowpass Filter/2, Varying Lowpass Filter1/2
  D/1 -> Sum1/3
  P/1 -> Sum1/2
  Derivative/1 -> D/1
  Integrator5/1 -> I/1
  MATLAB Function19/1(y) -> Scope28/1
  u/1 -> MATLAB Function19/2(u)
  v/1 -> MATLAB Function19/1(v)
  max rudder angle/1 -> MATLAB Function1/2(max), MATLAB Function/2(max)
  desired heading/1 -> Sum/2, Scope2/1, Sum2/1
  Sum2/1 -> Desired Heading/1
  Sum3/1 -> Scope4/1, P1/1
  Sum4/1 -> Scope5/1, Derivative1/1, Integrator1/1, P2/1
  Integrator1/1 -> I1/1
  Derivative1/1 -> D1/1
  D1/1 -> Sum5/3
  Varying Lowpass Filter1/1 -> MATLAB Function1/1(u)
  psi/1 -> Sum3/2, Sum/1
  D2/1 -> Scope3/1
  P1/1 -> desired yaw rate/1, Sum4/1
  r/1 -> Sum4/2
  I1/1 -> Scope6/1, Sum5/1
  P2/1 -> Scope7/1, Sum5/2
  Sum5/1 -> Varying Lowpass Filter1/1
  MATLAB Function1/1(y) -> rudder angle/1, D2/1, Scope1/2
  rudder step/1 -> Sum6/1
  MATLAB Function19/2(y1) -> Gain1/1, Gain12/1, Scope29/1, Sum6/2
  Sum6/1 -> Sum3/1

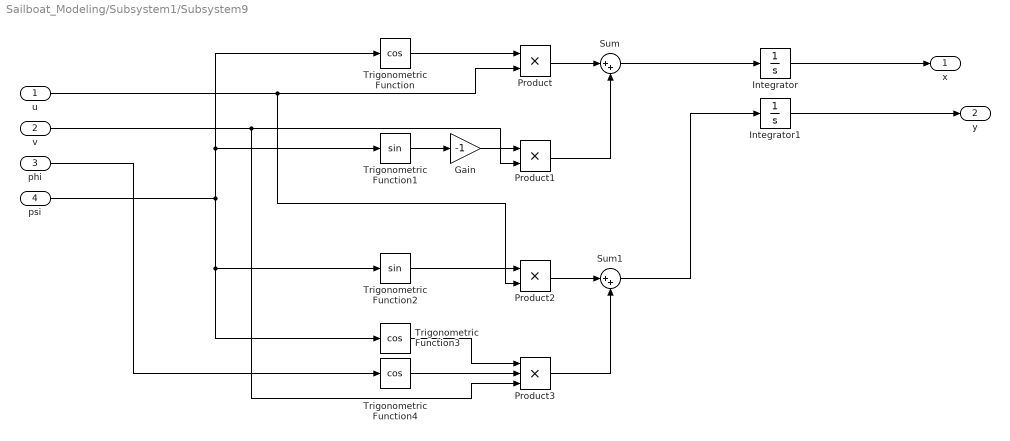
== system Sailboat_Modeling/Subsystem1/Subsystem9 ==
  u : Inport
  v : Inport  Port=2
  phi : Inport  Port=3
  psi : Inport  Port=4
  Gain : Gain  Gain=-1
  Integrator : Integrator
  Integrator1 : Integrator
  Product : Product
  Product1 : Product
  Product2 : Product
  Product3 : Product  Inputs=3
  Sum : Sum  Inputs=|++
  Sum1 : Sum  Inputs=|++
  Trigonometric Function : Trigonometry  Operator=cos
  Trigonometric Function1 : Trigonometry
  Trigonometric Function2 : Trigonometry
  Trigonometric Function3 : Trigonometry  Operator=cos
  Trigonometric Function4 : Trigonometry  Operator=cos
  x : Outport
  y : Outport  Port=2
  wires:
  Integrator/1 -> x/1
  Integrator1/1 -> y/1
  psi/1 -> Trigonometric Function1/1, Trigonometric Function/1, Trigonometric Function3/1, Trigonometric Function2/1
  Trigonometric Function/1 -> Product/1
  u/1 -> Product/2, Product2/2
  Trigonometric Function1/1 -> Gain/1
  Gain/1 -> Product1/1
  v/1 -> Product1/2, Product3/3
  Product/1 -> Sum/1
  Product1/1 -> Sum/2
  Sum/1 -> Integrator/1
  Product3/1 -> Sum1/2
  Sum1/1 -> Integrator1/1
  Trigonometric Function2/1 -> Product2/1
  Product2/1 -> Sum1/1
  Trigonometric Function3/1 -> Product3/1
  Trigonometric Function4/1 -> Product3/2
  phi/1 -> Trigonometric Function4/1

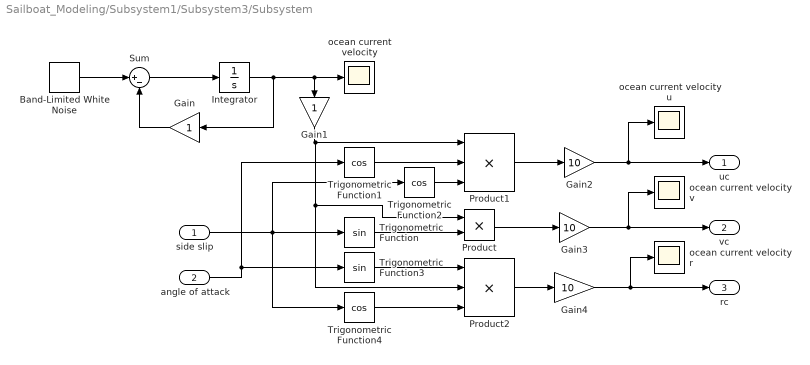
== system Sailboat_Modeling/Subsystem1/Subsystem3/Subsystem ==
  side slip : Inport
  angle of attack : Inport  Port=2
  Band-Limited White Noise : simulink/Sources/Band-Limited White Noise  Cov=[0.03]  Ts=1  seed=[23341]
  Gain : Gain
  Gain1 : Gain
  Gain2 : Gain  Gain=10
  Gain3 : Gain  Gain=10
  Gain4 : Gain  Gain=10
  Integrator : Integrator
  Product : Product
  Product1 : Product  Inputs=3
  Product2 : Product  Inputs=3
  Sum : Sum  Inputs=|+-
  Trigonometric Function : Trigonometry
  Trigonometric Function1 : Trigonometry  Operator=cos
  Trigonometric Function2 : Trigonometry  Operator=cos
  Trigonometric Function3 : Trigonometry
  Trigonometric Function4 : Trigonometry  Operator=cos
  ocean current velocity : Scope
  ocean current velocity r : Scope
  ocean current velocity u : Scope
  ocean current velocity v : Scope
  uc : Outport
  vc : Outport  Port=2
  rc : Outport  Port=3
  wires:
  Sum/1 -> Integrator/1
  Band-Limited White Noise/1 -> Sum/1
  Integrator/1 -> ocean current velocity/1, Gain1/1, Gain/1
  Gain/1 -> Sum/2
  Trigonometric Function/1 -> Product/2
  side slip/1 -> Trigonometric Function4/1, Trigonometric Function2/1, Trigonometric Function/1
  Product/1 -> Gain3/1
  Trigonometric Function2/1 -> Product1/3
  Trigonometric Function1/1 -> Product1/2
  Product1/1 -> Gain2/1
  Trigonometric Function3/1 -> Product2/1
  Trigonometric Function4/1 -> Product2/3
  angle of attack/1 -> Trigonometric Function3/1, Trigonometric Function1/1
  Product2/1 -> Gain4/1
  Gain1/1 -> Product1/1, Product2/2, Product/1
  Gain2/1 -> ocean current velocity u/1, uc/1
  Gain3/1 -> ocean current velocity v/1, vc/1
  Gain4/1 -> rc/1, ocean current velocity r/1

== matlab function Sailboat_Modeling/Subsystem1/MATLAB Function3 ==
  data: Xs output; delta_s input; wind_direction input; Ys output; Ks output; Ns output; awa output; wind_velocity input; psi input; u input; v input; r input; alpha_aw output; apparent_velocity output; V_awu output; V_awv output; L output; D output; rawa input; phi input; data output
function [Xs,Ys,Ks,Ns,awa,alpha_aw,apparent_velocity,V_awu,V_awv,L,D, data] = sailForce(delta_s,wind_direction,wind_velocity, psi, u, v,r,rawa,phi)
%Parameters
rho_a = 1.2;
area_sail =0.38;

% CoE of the sail
xs = 0;
ys = 0;
zs = 0.6;
xm = 0;
xsm = 0; 
v_t = [wind_velocity*cos(wind_direction); wind_velocity*sin(wind_direction); 0 ];
R1 = [ cos(-psi) -sin(-psi) 0; sin(-psi) cos(-psi) 0; 0 0 1];
R2 = [ 1 0 0 ; 0 1 0; 0 0 1];
v_tb = R2*R1*v_t; % wind expressed in the body frame
V_in = [ u ; v ; 0 ];
V_awb = v_tb - V_in ;
V_awu = V_awb(1);
V_awv = V_awb(2);
V_aw = V_awu^2 + V_awv^2;
alpha_aw = atan2(real(V_awv),real(-V_awu));


% Apparent Wind Velocity
awa=rawa;
apparent_velocity = sqrt(V_aw);

% Calculate Angle of Attack
%alpha = awa+delta_s;
alpha = awa + delta_s;
data = delta_s;
%ds = -0.5*awa;
% Calculate Lift and Drag Force
[Cls,Cds] = sailcoef(alpha);
Ls = 0.5*rho_a*area_sail*(apparent_velocity)^2*Cls;
Ds = 0.5*rho_a*area_sail*(apparent_velocity)^2*Cds;

% Sail Force components
Xs =(Ls * sin(awa) - Ds * cos(awa))*cos(phi);
Ys = (Ls * cos(awa) + Ds * sin(awa));
Ks = -zs *(Ls * cos(awa) + Ds * sin(awa))*cos(phi);
Ns = (-Xs * xsm * sin(delta_s) +Ys*(xm-xsm*cos(delta_s)));
L = Ls*sin(awa);
D = -Ds*cos(awa);

function [Cls,Cds] = sailcoef(attack)
% generate a lookup table for the lift/drag coefficients for the sail
% and compute Cls/Cds from the lookup table using interpolation.

% lookup table
xdata = linspace(-pi,pi,73); % every 5 degrees
xdata = xdata/pi*180;

% lift curve
yldata = [fliplr([0 0.15 0.32 ...
    0.48 0.7 0.94 1.15 1.3 1.28 1.15 1.1 1.05 1 0.9 0.82 0.72 0.68 0.56 0.48 0.32 0.21 0.08 ...
    -0.06 -0.18 -0.3 -0.4 -0.53 -0.64 -0.72 -0.84 -0.95 -1.04 -1.1 -1.14 -1.08 -0.76 0])*(-1) ...
    [0.15 0.32 ...
    0.48 0.7 0.94 1.15 1.3 1.28 1.15 1.1 1.05 1 0.9 0.82 0.72 0.68 0.56 0.48 0.32 0.21 0.08 ...
    -0.06 -0.18 -0.3 -0.4 -0.53 -0.64 -0.72 -0.84 -0.95 -1.04 -1.1 -1.14 -1.08 -0.76 0]];

% drag curve
yddata = [fliplr([0.1 0.12 0.14 ...
    0.16 0.19 0.26 0.35 0.46 0.54 0.62 0.7 0.78 0.9 0.98 1.04 1.08 1.16 1.2 1.24 1.26 ...
    1.28 1.34 1.36 1.37 1.33 1.31 1.28 1.26 1.25 1.2 1.1 1.04 0.88 0.8 0.64 0.38 0.1])...
    [0.12 0.14 ...
    0.16 0.19 0.26 0.35 0.46 0.54 0.62 0.7 0.78 0.9 0.98 1.04 1.08 1.16 1.2 1.24 1.26 ...
    1.28 1.34 1.36 1.37 1.33 1.31 1.28 1.26 1.25 1.2 1.1 1.04 0.88 0.8 0.64 0.38 0.1]];

% fit the input angle of attack into the interval [-pi,pi]
if attack > pi
    attack = mod(attack+pi,2*pi) - pi;
else
    if attack < -pi
        attack = mod(attack-pi,-2*pi) + pi;
    end
end

% interpolation
attack = attack/pi*180;
Cls = interp1(xdata,yldata,attack,'pchip');
Cds = interp1(xdata,yddata,attack,'pchip');

== matlab function Sailboat_Modeling/Subsystem1/MATLAB Function4 ==
  data: r input; u input; Xr output; v input; Yr output; Kr output; Nr output; delta_r input; delta_r output; alpha_a output; p input; phi input; lift_force output; drag_force output
function [Xr, Yr, Kr, Nr, delta_r, alpha_a, lift_force, drag_force] = rudderForce(r, u, v, delta_r, p, phi)
%Parameters
rudder_width = 4;
rudder_length = 20;
rho_w = 1025;
area = rudder_length * rudder_width * 10^(-4);
velocity = sqrt(v^2+u^2);
yr = 0;
xr = 0.55;
zr = 0.2;
zeta_r =1; % Rudder Efficiency
d_r = 0.2; % Rudder Draft
% Calculate Angle of Attack
v_aru = -u + r*yr;
v_arv = -v-r*xr;
alpha_ar = atan2(real(v_arv),real(v_aru));
alpha_a = alpha_ar - delta_r;

% Lift and Drag Coeff
[lc, dc] = ruddercoef(alpha_a);
dc = dc+lc^2*area*(pi*2*zeta_r*d_r^2);

% Calculate Lift and Drag Force
lift_force = 0.5 * rho_w * area * lc * (v_aru^2+v_arv^2) ;
drag_force = 0.5 * rho_w * area * dc * (v_aru^2+v_arv^2) ;

Xr = (lift_force * sin(alpha_ar) - drag_force * cos(alpha_ar));
Yr = (lift_force * cos(alpha_ar) + drag_force * sin(alpha_ar))*cos(phi);
Kr = zr * ( -lift_force * cos(alpha_ar) - drag_force * sin(alpha_ar));
Nr = xr * (lift_force * cos(alpha_ar) + drag_force * sin(alpha_ar))*cos(phi);
Nr = Nr*1.25;


function [Clr,Cdr] = ruddercoef(attack)
% generate a lookup table for the lift/drag coefficients for the sail
% and compute Cls/Cds from the lookup table using interpolation.

% lookup table
xdata = linspace(-pi,pi,73); % every 5 degrees
xdata = xdata/pi*180;

% lift curve
yl = fliplr([0 0.42 0.73 ...
    0.95 1.1 1.165 1.18 1.155 1.12 1.065 1 0.92 0.83 0.72 0.62 0.48 0.33 0.16])*(-1);
yldata = [fliplr([0 0.42 0.73 ...
    0.95 1.1 1.165 1.18 1.155 1.12 1.065 1 0.92 0.83 0.72 0.62 0.48 0.33 0.16 0 yl])*(-1) ...
    [0.42 0.73 ...
    0.95 1.1 1.165 1.18 1.155 1.12 1.065 1 0.92 0.83 0.72 0.62 0.48 0.33 0.16 0 yl]];

% drag curve
yd = fliplr([0 0.03 0.06 ...
    0.1 0.17 0.3 0.48 0.74 0.98 1.18 1.34 1.5 1.65 1.76 1.89 1.97 2.01 2.05]);
yddata = [fliplr([0 0.03 0.06 ...
    0.1 0.17 0.3 0.48 0.74 0.98 1.18 1.34 1.5 1.65 1.76 1.89 1.97 2.01 2.05 2.08 yd])...
    [0.03 0.06 ...
    0.1 0.17 0.3 0.48 0.74 0.98 1.18 1.34 1.5 1.65 1.76 1.89 1.97 2.01 2.05 2.08 yd]];

% fit the input angle of attack into the interval [-pi,pi]
if attack > pi
    attack = mod(attack+pi,2*pi) - pi;
else
    if attack < -pi
        attack = mod(attack-pi,-2*pi) + pi;
    end
end

% interpolation
attack = attack/pi*180;
Clr = interp1(xdata,yldata,attack,'pchip');
Cdr = interp1(xdata,yddata,attack,'pchip');

== matlab function Sailboat_Modeling/Subsystem1/MATLAB Function5 ==
  data: r input; u input; Xk output; v input; Yk output; Kk output; Nk output; phi input
function [Xk,Yk,Kk,Nk] = keelForce(r,u,v,phi)
%Parameters
keel_width = 8;
keel_length = 45;
rho_w = 1025;
area = keel_width * keel_length * 10^(-4);
velocity = sqrt(v^2+u^2);
l3 = 0.1;
h2 =0.275;
yk=0;
xk=0;
zk=0.25;
zeta_r = 1;
d_r = 0.4;
% Calculate Angle of Attack
v_aku = -u + r*yk;
v_akv = -v - r*xk + 0*zk;
alpha_ak = atan2(real(v_akv),real(-v_aku));
alpha = alpha_ak;

% Lift and Drag Coeff
[lc, dc] = keelcoef(alpha);
dc = dc+lc^2*area*(pi*2*zeta_r*d_r^2);

% Calculate Lift and Drag Force
lift_force = 0.5 * rho_w * area * lc * (v_aku^2+v_akv^2);
drag_force = 0.5 * rho_w * area * dc * (v_aku^2+v_akv^2);

Xk = (-lift_force * sin(alpha_ak) + drag_force * cos(alpha_ak));
Yk = (-lift_force * cos(alpha_ak) - drag_force * sin(alpha_ak))*cos(phi);
Kk = (lift_force*cos(alpha_ak)+drag_force*sin(alpha_ak))*zk;
Nk = (-(lift_force*cos(alpha_ak)-drag_force*sin(alpha_ak))*xk)*cos(phi);




%------------------------------------------------------------------------------------------------------------------------------
function [Clk,Cdk] = keelcoef(attack)
% generate a lookup table for the lift/drag coefficients for the sail
% and compute Cls/Cds from the lookup table using interpolation.

% lookup table
xdata = linspace(-pi,pi,73); % every 5 degrees
xdata = xdata/pi*180;

% lift curve
yl = fliplr([0 0.425 0.74 ...
    0.94 1.1 1.17 1.19 1.16 1.12 1.07 0.99 0.92 0.84 0.74 0.63 0.49 0.345 0.185])*(-1);
yldata = [fliplr([0 0.425 0.74 ...
    0.94 1.1 1.17 1.19 1.16 1.12 1.07 0.99 0.92 0.84 0.74 0.63 0.49 0.345 0.185 0 yl])*(-1) ...
    [0.425 0.74 ...
    0.94 1.1 1.17 1.19 1.16 1.12 1.07 0.99 0.92 0.84 0.74 0.63 0.49 0.345 0.185 0 yl]];

% drag curve
yd = fliplr([0 0.04 0.07 ...
    0.1 0.17 0.3 0.49 0.76 0.98 1.19 1.34 1.5 1.65 1.77 1.88 1.96 2.01 2.05]);
yddata = [fliplr([0 0.04 0.07 ...
    0.1 0.17 0.3 0.49 0.76 0.98 1.19 1.34 1.5 1.65 1.77 1.88 1.96 2.01 2.05 2.09 yd])...
    [0.04 0.07 ...
    0.1 0.17 0.3 0.49 0.76 0.98 1.19 1.34 1.5 1.65 1.77 1.88 1.96 2.01 2.05 2.09 yd]];

% fit the input angle of attack into the interval [-pi,pi]
if attack > pi
    attack = mod(attack+pi,2*pi) - pi;
else
    if attack < -pi
        attack = mod(attack-pi,-2*pi) + pi;
    end
end

% interpolation
attack = attack/pi*180;
Clk = interp1(xdata,yldata,attack,'pchip');
Cdk = interp1(xdata,yddata,attack,'pchip');


%------------------------------------------------------------------------------------------------------------------------------
function F = resistancehull(alpha_a)

xdata = linspace(0,6,13); % every 0.5m/s
ydata = [0 0.15 0.35 0.5 0.675 0.825 1.175 1.4 2 4.85 9.85 18.46 27.5]*1000;

% interpolation
if alpha_a <= 6
    F = interp1(xdata,ydata,alpha_a,'pchip');
else
    F = interp1(xdata,ydata,alpha_a,'pchip','extrap');
end

== matlab function Sailboat_Modeling/Subsystem1/MATLAB Function6 ==
  data: r input; u input; Xh output; v input; Yh output; Kh output; Nh output; Frh output; phi input; alpha_ah output
function [Xh,Yh,Kh,Nh,Frh,alpha_ah] = hullForce(r,u,v,phi)
yh = 0;
zh = 0.1;
xh = 0;
B = 0.125;
rho = 1025;
L = 0.95;
Lwl =0.85;
g = 9.81;
delta =  4*pi * (((0.475*0.0625)^(1.6)+(0.475*0.1)^(1.6)+(0.0625*0.1)^(1.6))/(3))^(1/1.6);
% from the hull
v_ahu = -u + r*yh;
v_ahv = (-v-r*xh + 0*zh)/cos(0);
v_ah = sqrt(v_ahu^2 + v_ahv^2);
alpha_ah = atan2(real(v_ahv),real(v_ahu));
%Frh = resistancehull(u);
Re = (abs(v_ahu)*Lwl)/(0.00000010034);
Cf = 0.075 / (log(Re)-2)^2;
Frh = 0.5 * rho * u^2 * Cf * (delta);

Xh = Frh;

Yh = -Frh*sin(alpha_ah)*cos(phi);

if abs(Yh)>15
    if Yh >0
        Yh=15;
    else
        Yh = -15;
    end
end
Kh = Frh*sin(alpha_ah)*cos(phi)*zh;

if abs(Kh)>15
    if Kh >0
        Kh=15;
    else
        Kh = -15;
    end
end
Nh = -Frh*sin(alpha_ah)*cos(0)*xh;
%D_hull = [Frh*cos(alpha_ah);-Frh*sin(alpha_ah)*cos(phi); Frh*sin(alpha_ah)*cos(phi)*par.zh; -Frh*sin(alpha_ah)*cos(phi)*par.xh];


function F = resistancehull(alpha_a)

xdata = linspace(0,2.6,13); % every 0.5m/s
ydata = [0 6.0018e-04 0.0039*0.0039 0.0127*0.0127 0.0306*0.0306 0.0625*0.0625 0.1157*0.1157 0.2002*0.2002 0.3304*0.3304 0.5274*0.5274 0.8219*0.8 1.2606*0.9 1.9151];

% interpolation
if alpha_a <= 1.3
    F = interp1(xdata,ydata,alpha_a,'pchip');
else
    F = interp1(xdata,ydata,alpha_a,'pchip','extrap');
end

== matlab function Sailboat_Modeling/Subsystem1/Subsystem8/MATLAB Function19 ==
  data: y output; v input; u input; y1 output
function [y,y1]     = beta(v,u)
% Beta Reference Angle
y=0;
y1 = real(asin(complex(v/sqrt(v^2+u^2))));

== matlab function Sailboat_Modeling/Subsystem1/Subsystem7/MATLAB Function1 ==
  data: roll_angle input; current_state input; t input; sail_angle output; t_prev input; next_state output; t_state_change output; apparent_wind_angle input
%%%%%%%%%%%%%%%%%%%%%%%%%%%%%%%%%%%%%%%%%%%%%%%%%%%%%%%%%%%%%%
%SAIL CONTROLLER
%%%%%%%%%%%%%%%%%%%%%%%%%%%%%%%%%%%%%%%%%%%%%%%%%%%%%%%%%%%%%%
function [sail_angle,next_state,t_state_change]  = sailAngle(roll_angle,current_state,t,t_prev,apparent_wind_angle)
switch(current_state)
    case 0
        sail_angle = 15;
            if abs(roll_angle) <15
               next_state = 1;
               t_state_change = t;
            else
                next_state =0;
                t_state_change = t_prev;
            end
    case 1
        sail_angle = 15/7 * roll_angle + 17.14;
            if abs(roll_angle) > 15
                next_state = 0;
                t_state_change = t;
            elseif abs(roll_angle) <8
                next_state =2;
                t_state_change = t;
            else
                next_state =1;
                t_state_change = t_prev;
            end
    case 2
        sail_angle = 0;
            if abs(roll_angle) > 8
                next_state = 1;
                t_state_change = t;
            else 
                next_state =2;
                t_state_change = t_prev;
            end
    otherwise
        sail_angle = 60;
        next_state=0;
        t_state_change = t;
end
if apparent_wind_angle >0 
    sail_angle = -sail_angle;
end

== matlab function Sailboat_Modeling/Subsystem1/Subsystem2/MATLAB Function ==
  data: u input; y output
function y = fcn(u)
if u>0
    y = -0.035
else 
    y=0;
end

== matlab function Sailboat_Modeling/Subsystem1/Subsystem7/MATLAB Function2 ==
  data: delta_s input; y output; awa input
function y = fcn(delta_s,awa)
if awa>0
    y=-delta_s;
else 
    y= delta_s;
end

== matlab function Sailboat_Modeling/Subsystem1/Subsystem7/MATLAB Function3 ==
  data: y output; awa input
function y = fcn(awa)
if awa>0
    y=-8;
else 
    y= 8;
end

== matlab function Sailboat_Modeling/Subsystem1/Subsystem8/MATLAB Function ==
  data: u input; y output; max input
function y = fcn(u,max)
if u>max
    u=max;
else 
    if u<-max
        u=-max;
    end
end
y = u;

== matlab function Sailboat_Modeling/Subsystem1/Subsystem7/MATLAB Function ==
  data: u input; y output; max input; min input
function y = fcn(u,max,min)
if u>max
    u=max;
else 
    if u<min
        u=min;
    end
end
if u<0
 u=-u;
end
y = u;

== matlab function Sailboat_Modeling/Subsystem1/Subsystem8/MATLAB Function1 ==
  data: u input; y output; max input
function y = fcn(u,max)
if u>max
    u=max;
else 
    if u<-max
        u=-max;
    end
end
y = u;

== matlab function Sailboat_Modeling/Subsystem1/Subsystem3/MATLAB Function14 ==
  data: beta input; wu output; wv output; wr output; t input
function [wu,wv,wr] = WaveForcesandMoments(beta,t)
% Water density (kg/m^2)
rho = 1025;

% Gravity (m/s^2)
g = 9.81;

% Vessel size (m)
L = 1;
B = 0.125;
T = 0.4;

% Vessels Heading

% Wave Specifications
% amplitude(m)
Ai = 2;
% length(m)
lamdai = 1;
% encounter frequency (rads)
omegai = 0.4;
% random phase (rads)
phii = -pi;

% Wave Component
waveC = Ai * (2*pi)/lamdai * sin(omegai*t + phii);

% u Component
wu = (10^(-6)) * rho * g * B * L * T * cos(beta) * waveC;

% v Component
wv = (10^(-6)) * rho * g * B * L * T * sin(beta) * waveC;

% r Component
wr = (10^(-6)) * 1/24 * rho * g * B * L * (L^2 - B^2) * sin(2*beta) * waveC^2;

== matlab function Sailboat_Modeling/Subsystem1/Subsystem3/MATLAB Function15 ==
  data: windDirect input; wi_u output; wi_v output; wi_r output; V_w input; psi input; u input; v input
function [wi_u,wi_v,wi_r] = WindForcesandMoments(windDirect,V_w,psi,u,v)
% Air density (kg/m^2)
rho = 1.225;

% Ship Size
L = 2;
B = 0.125;
T = 0.4;

% centroids above the water line of the frontal and lateral projected areas
H_fw = T - 1.2;
H_lw = T - 1.2;
A_fw = B * H_fw;
A_lw = L * H_lw;


% Symmetrical Ship Coeff
c_x = 0.7;
c_y = 0.825;
c_r = 0.125;

% Wind Velocities in x- and y-coordinates
u_w = V_w * cos(windDirect - psi);
v_w = V_w * sin(windDirect - psi);

% Relative wind velocities
u_rw = u - u_w;
v_rw = v - v_w;

% Relative Wind Velocity and direction
V_rw = sqrt(u_rw^2 + v_rw^2);
gamma_rw = -atan(v_rw/u_rw);

% Wind Coeff
C_x = -c_x * cos(gamma_rw);
C_y = c_y * sin(gamma_rw);
C_r = c_r * sin(2*gamma_rw);

% Wind Forces and Moments
wi_u = 0.5 * rho * V_rw *  C_x * A_fw * 10^(-2);
wi_v = 0.5 * rho * V_rw *  C_y * A_lw * 10^(-2);
wi_r = 0.5 * rho * V_rw *  C_r * A_lw * 10^(-2);
